simulink model "mask_control_struct"  (R2013b)
settings: Solver=ode45  StartTime=0.0  StopTime=10.0  RelTol=1e-3
settings Model: Creator=Administrator  LastModifiedBy=Administrator

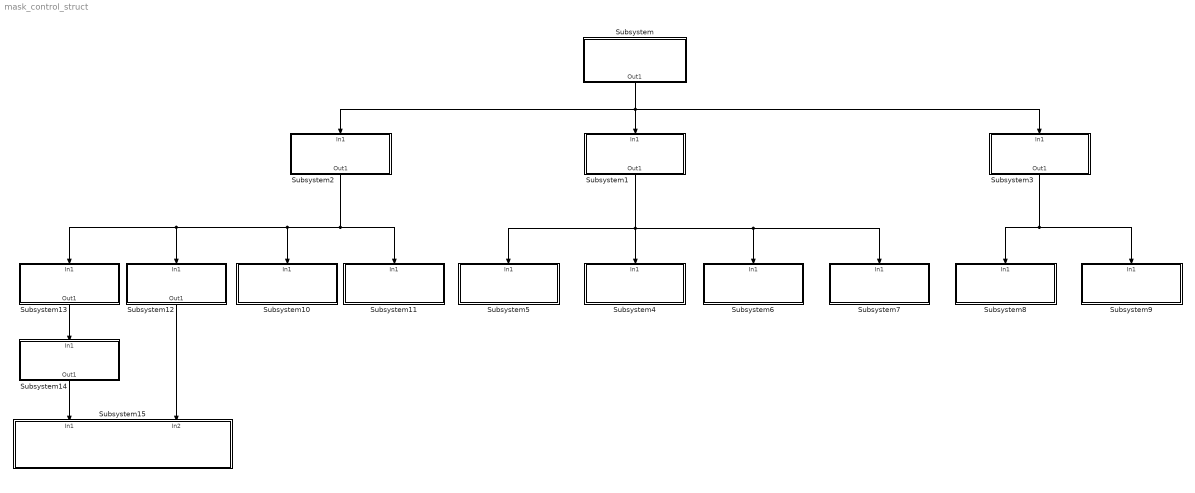
== system mask_control_struct ==
  Subsystem : Subsystem
      mask Display: disp('Mask Control');
  Subsystem1 : Subsystem
      mask Display: disp('Parameter');
  Subsystem10 : Subsystem
      mask Display: disp('text');
  Subsystem11 : Subsystem
      mask Display: disp('image');
  Subsystem12 : Subsystem
      mask Display: disp('groupbox');
  Subsystem13 : Subsystem
      mask Display: disp('tabcontainer');
  Subsystem14 : Subsystem
      mask Display: disp('tab');
  Subsystem15 : Subsystem
      mask Display: disp('Sub Mask Control');
  Subsystem2 : Subsystem
      mask Display: disp('Display');
  Subsystem3 : Subsystem
      mask Display: disp('Action');
  Subsystem4 : Subsystem
      mask Display: disp('edit');
  Subsystem5 : Subsystem
      mask Display: disp('checkbox');
  Subsystem6 : Subsystem
      mask Display: disp('radiobutton');
  Subsystem7 : Subsystem
      mask Display: disp('popupmenu');
  Subsystem8 : Subsystem
      mask Display: disp('hyperlink');
  Subsystem9 : Subsystem
      mask Display: disp('pushbutton');
  wires:
  Subsystem/1(Out1) -> Subsystem3/1(In1), Subsystem2/1(In1), Subsystem1/1(In1)
  Subsystem1/1(Out1) -> Subsystem7/1(In1), Subsystem6/1(In1), Subsystem5/1(In1), Subsystem4/1(In1)
  Subsystem3/1(Out1) -> Subsystem9/1(In1), Subsystem8/1(In1)
  Subsystem2/1(Out1) -> Subsystem13/1(In1), Subsystem12/1(In1), Subsystem10/1(In1), Subsystem11/1(In1)
  Subsystem13/1(Out1) -> Subsystem14/1(In1)
  Subsystem14/1(Out1) -> Subsystem15/1(In1)
  Subsystem12/1(Out1) -> Subsystem15/2(In2)

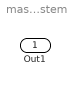
== system mask_control_struct/Subsystem ==
  Out1 : Outport

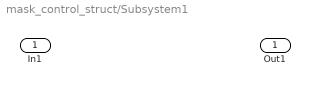
== system mask_control_struct/Subsystem1 ==
  In1 : Inport
  Out1 : Outport

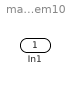
== system mask_control_struct/Subsystem10 ==
  In1 : Inport

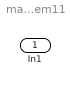
== system mask_control_struct/Subsystem11 ==
  In1 : Inport

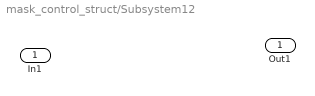
== system mask_control_struct/Subsystem12 ==
  In1 : Inport
  Out1 : Outport

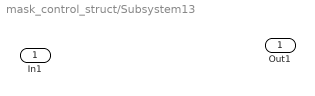
== system mask_control_struct/Subsystem13 ==
  In1 : Inport
  Out1 : Outport

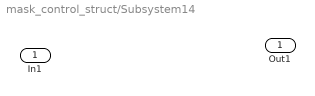
== system mask_control_struct/Subsystem14 ==
  In1 : Inport
  Out1 : Outport

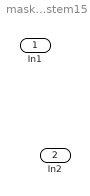
== system mask_control_struct/Subsystem15 ==
  In1 : Inport
  In2 : Inport  Port=2

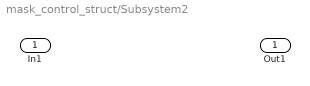
== system mask_control_struct/Subsystem2 ==
  In1 : Inport
  Out1 : Outport

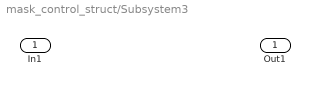
== system mask_control_struct/Subsystem3 ==
  In1 : Inport
  Out1 : Outport

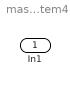
== system mask_control_struct/Subsystem4 ==
  In1 : Inport

== system mask_control_struct/Subsystem5 ==
  In1 : Inport

== system mask_control_struct/Subsystem6 ==
  In1 : Inport

== system mask_control_struct/Subsystem7 ==
  In1 : Inport

== system mask_control_struct/Subsystem8 ==
  In1 : Inport

== system mask_control_struct/Subsystem9 ==
  In1 : Inport
